simulink model "los_test_with_camsim_kalman2"  (Simulink 7.1)
settings: Solver=ode5  StartTime=0.0  StopTime=700  FixedStep=0.1  RelTol=1e-3
values from neighbouring files (symbols this model uses):
  bottom = u(7)    [camsim.m]    (also in camsim2.m = u(13); camsim3.m = u(13); ekf2.m = u(31); initauv.m = 4)
undefined symbols (not defined in the file or in its folder): ekf2
libraries: fordypningsprosjekt x3, simulink x1
settings Model: Creator=anderga  LastModifiedBy=anders

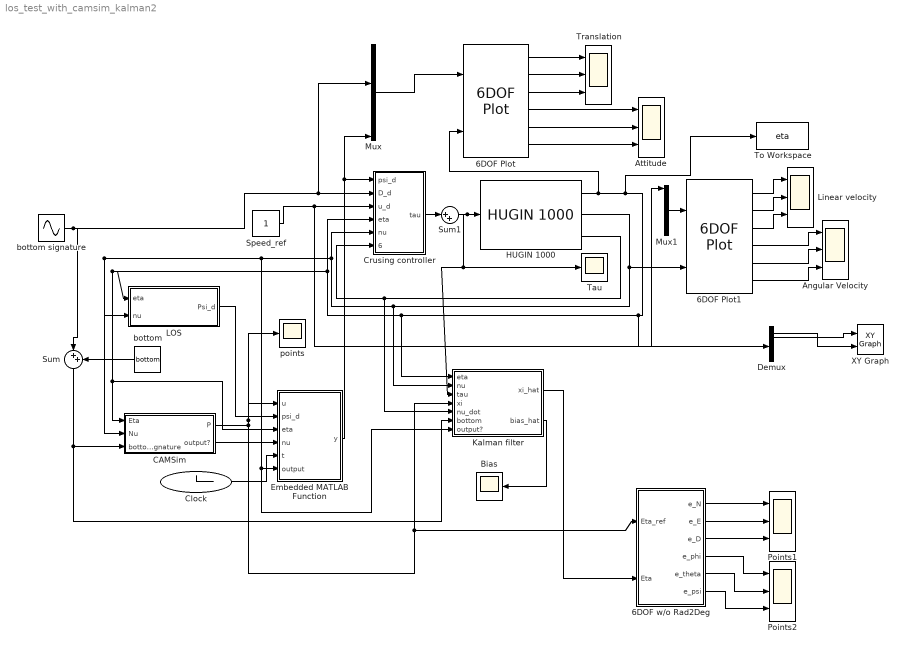
== system los_test_with_camsim_kalman2 ==
  6DOF Plot : fordypningsprosjekt/6DOF Plot  SystemSampleTime=-1
  6DOF Plot1 : fordypningsprosjekt/6DOF Plot  SystemSampleTime=-1
  6DOF w/o Rad2Deg : Subsystem  AncestorBlock=fordypningsprosjekt/6DOF Plot
      mask Type: 6 DOF plot reference versus eta
  Angular Velocity : Scope  NumInputPorts=3
      settings: YMin=-5~0~-40  YMax=5~0.3~40  SaveName=ScopeData3
  Attitude : Scope  NumInputPorts=3
      settings: YMin=-0.2~0~-200  YMax=0.25~0.5~200  SaveName=Attitude_ref
  Bias : Scope
      settings: YMin=-1  YMax=1  SaveName=Camsim_output1  DataFormat=Array
  CAMSim : Subsystem  AncestorBlock=fordypningsprosjekt/CAMSim
  Clock : Clock
  Crusing controller : Subsystem  AncestorBlock=fordypningsprosjekt/Crusing controller  mask{Kp_u=10, Ki_u=3, Kp_c=100, Kd_c=50, Kp_d=50, Kp2_d=20, Kd_d=20}
      mask prompts: Kp_u "Kp Speed controller"; Ki_u "Ki Speed Controller"; Kp_c "Kp Course Controller"; Kd_c "Kd Course Controller"; Kp_d "Kp1 Depth Controller"; Kp2_d "Kp2 Depth controller"; Kd_d "Kd Depth Controller"
  Demux : Demux  Outputs=6
  Embedded MATLAB Function : Stateflow chart
  HUGIN 1000 : fordypningsprosjekt/HUGIN 1000  SystemSampleTime=-1  eta_0=eta0  nu_0=[0 0 0 0 0 0]  c_on_off=off  beta_c=45  V_c=0.5
  Kalman filter : Subsystem  AncestorBlock=fordypningsprosjekt/Kalman filter
  LOS : Subsystem
  Linear velocity : Scope  NumInputPorts=3
      settings: YMin=0.5~-1.25~-0.125  YMax=1.9~0.75~0  SaveName=Lin_veloc
  Mux : Mux  Inputs=6
  Mux1 : Mux  Inputs=6
  Points1 : Scope  NumInputPorts=3
      settings: YMin=-1.75~-0.5~-1.75  YMax=0.5~0.5~0.5  SaveName=Translation_ref1
  Points2 : Scope  NumInputPorts=3
      settings: TimeRange=700  YMin=-0.4~-1.25~-0.5  YMax=0.5~0.5~0.5  SaveName=Attitude_ref1
  Speed_ref : Constant  OutDataType=sfix(16)  OutScaling=2^0
  Sum : Sum  Orientation=down  Inputs=|++  OutDataType=sfix(16)  OutScaling=2^0
  Sum1 : Sum  Inputs=|++  OutDataType=sfix(16)  OutScaling=2^0
  Tau : Scope
      settings: TimeRange=700  YMin=-5500  YMax=3000  SaveName=ScopeData4
  To Workspace : ToWorkspace  VariableName=eta  SampleTime=-1  SaveFormat=Structure With Time
  Translation : Scope  NumInputPorts=3
      settings: YMin=0~-125~0  YMax=125~0~60  SaveName=Translation_ref
  XY Graph : simulink/Sinks/XY Graph  SystemSampleTime=-1  xmin=-100  xmax=100  ymin=-100  ymax=500  st=-1
  bottom : Constant  Orientation=left  Value=bottom  OutDataType=sfix(16)  OutScaling=2^0
  bottom signature : Sin  Amplitude=6  Bias=50  Frequency=0.01  SampleTime=0
  points : Scope
      settings: TimeRange=500  YMin=-0.035  YMax=0.035  SaveName=Camsim_output  DataFormat=Array
  wires:
  HUGIN 1000/1 -> 6DOF Plot/2, Demux/1, Crusing controller/4(eta), LOS/1(eta), CAMSim/1(Eta), Embedded MATLAB Function/3(eta), Kalman filter/1(eta), To Workspace/1
  HUGIN 1000/2 -> 6DOF Plot1/2, Crusing controller/5(nu), LOS/2(nu), CAMSim/2(Nu), Embedded MATLAB Function/4(nu), Kalman filter/2(nu)
  HUGIN 1000/3 -> Crusing controller/6(nu_dot), Kalman filter/5(nu_dot)
  bottom signature/1 -> Crusing controller/2(D_d), Mux/3, Sum/1
  Speed_ref/1 -> Crusing controller/3(u_d), Mux1/1
  Mux/1 -> 6DOF Plot/1
  6DOF Plot/1 -> Translation/1
  6DOF Plot/2 -> Translation/2
  6DOF Plot/3 -> Translation/3
  6DOF Plot/4 -> Attitude/1
  6DOF Plot/5 -> Attitude/2
  6DOF Plot/6 -> Attitude/3
  Mux1/1 -> 6DOF Plot1/1
  6DOF Plot1/1 -> Linear velocity/1
  6DOF Plot1/2 -> Linear velocity/2
  6DOF Plot1/3 -> Linear velocity/3
  6DOF Plot1/4 -> Angular Velocity/1
  6DOF Plot1/5 -> Angular Velocity/2
  6DOF Plot1/6 -> Angular Velocity/3
  Demux/1 -> XY Graph/2
  Demux/2 -> XY Graph/1
  Sum/1 -> CAMSim/3(bottom_signature), Kalman filter/6(bottom)
  bottom/1 -> Sum/2
  Embedded MATLAB Function/1(y) -> Crusing controller/1(psi_d), Mux/6
  LOS/1(Psi_d) -> Embedded MATLAB Function/2(psi_d)
  CAMSim/1(P) -> Embedded MATLAB Function/1(u), points/1, 6DOF w/o Rad2Deg/1(Eta_ref), Kalman filter/4(xi)
  Clock/1 -> Embedded MATLAB Function/5(t)
  Kalman filter/1(xi_hat) -> 6DOF w/o Rad2Deg/2(Eta)
  6DOF w/o Rad2Deg/1(e_N) -> Points1/1
  6DOF w/o Rad2Deg/2(e_E) -> Points1/2
  6DOF w/o Rad2Deg/3(e_D) -> Points1/3
  6DOF w/o Rad2Deg/4(e_phi) -> Points2/1
  6DOF w/o Rad2Deg/5(e_theta) -> Points2/2
  6DOF w/o Rad2Deg/6(e_psi) -> Points2/3
  Kalman filter/2(bias_hat) -> Bias/1
  Crusing controller/1(tau) -> Sum1/1
  Sum1/1 -> HUGIN 1000/1, Tau/1, Kalman filter/3(tau)
  CAMSim/2(output?) -> Embedded MATLAB Function/6(output), Kalman filter/7(output?)

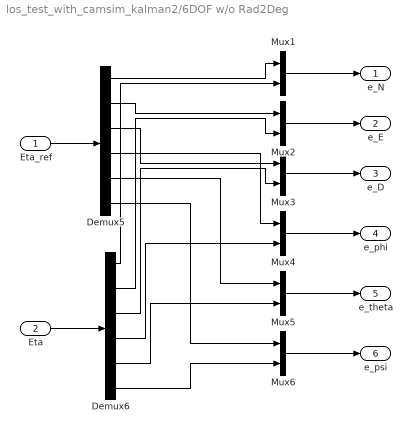
== system los_test_with_camsim_kalman2/6DOF w/o Rad2Deg ==
  Eta_ref : Inport  OutDataType=sfix(16)  OutScaling=2^0
  Eta : Inport  Port=2  OutDataType=sfix(16)  OutScaling=2^0
  Demux5 : Demux  Outputs=6
  Demux6 : Demux  Outputs=6
  Mux{1..6} (6 alike) : Mux  Inputs=2
  e_N : Outport  OutDataType=sfix(16)  OutScaling=2^0
  e_E : Outport  Port=2  OutDataType=sfix(16)  OutScaling=2^0
  e_D : Outport  Port=3  OutDataType=sfix(16)  OutScaling=2^0
  e_phi : Outport  Port=4  OutDataType=sfix(16)  OutScaling=2^0
  e_theta : Outport  Port=5  OutDataType=sfix(16)  OutScaling=2^0
  e_psi : Outport  Port=6  OutDataType=sfix(16)  OutScaling=2^0
  wires:
  Demux5/1 -> Mux1/1
  Demux6/1 -> Mux1/2
  Demux5/2 -> Mux2/1
  Demux5/3 -> Mux3/1
  Demux6/2 -> Mux2/2
  Demux6/3 -> Mux3/2
  Eta/1 -> Demux6/1
  Mux1/1 -> e_N/1
  Mux2/1 -> e_E/1
  Mux3/1 -> e_D/1
  Mux4/1 -> e_phi/1
  Mux5/1 -> e_theta/1
  Mux6/1 -> e_psi/1
  Demux5/4 -> Mux4/1
  Demux6/4 -> Mux4/2
  Demux5/5 -> Mux5/1
  Demux6/5 -> Mux5/2
  Demux6/6 -> Mux6/2
  Demux5/6 -> Mux6/1
  Eta_ref/1 -> Demux5/1

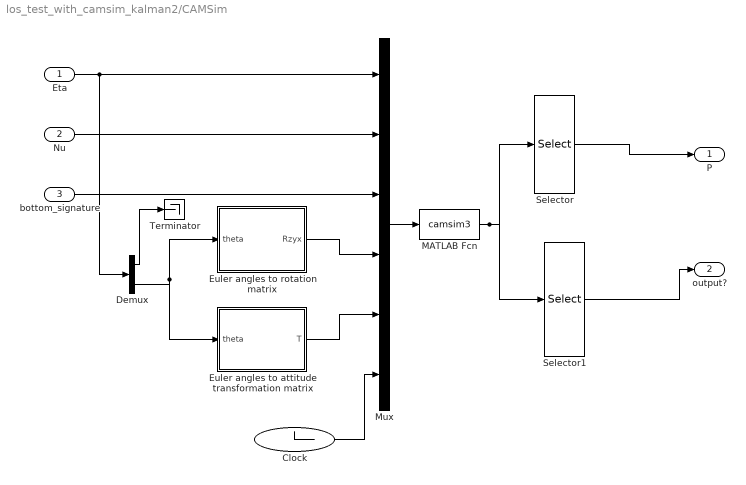
== system los_test_with_camsim_kalman2/CAMSim ==
  Eta : Inport  OutDataType=sfix(16)  OutScaling=2^0
  Nu : Inport  Port=2  OutDataType=sfix(16)  OutScaling=2^0
  bottom_signature : Inport  Port=3  OutDataType=sfix(16)  OutScaling=2^0
  Clock : Clock
  Demux : Demux  Outputs=2
  Euler angles to rotation matrix : Subsystem  AncestorBlock=marine_gnc/Models/ Kinematics/Euler angles to rotation matrix
      mask Type: Euler2R
      mask Description:
      | Determine the 3-by-3 rotation matrix from the Euler angles (roll, pitch, yaw) using the zyx convention.
      | 
      | Output is a 9x1 vector
      mask Display:
      | port_label('input',1,'theta')
      | port_label('output',1,'R')
  Euler angles to attitude transformation matrix : Subsystem  AncestorBlock=marine_gnc/Models/ Kinematics/Euler angles to attitude transformation matrix
      mask Type: Euler2T
      mask Description: Determine the 3-by-3 attitude transformation matrix  from the Euler angles (roll, pitch, yaw).
      mask Display:
      | port_label('input',1,'theta')
      | port_label('output',1,'T')
  MATLAB Fcn : MATLABFcn  MATLABFcn=camsim3  OutputDimensions=7
  Mux : Mux  Inputs=6
  Selector : Selector  InputPortWidth=7  IndexOptions=Index vector (dialog)  Indices=[1 2 3 4 5 6]  OutputSizes=1
  Selector1 : Selector  InputPortWidth=7  IndexOptions=Index vector (dialog)  Indices=[7]  OutputSizes=1
  Terminator : Terminator
  P : Outport  OutDataType=sfix(16)  OutScaling=2^0
  output? : Outport  Port=2  OutDataType=sfix(16)  OutScaling=2^0
  wires:
  Eta/1 -> Mux/1, Demux/1
  Nu/1 -> Mux/2
  bottom_signature/1 -> Mux/3
  Mux/1 -> MATLAB Fcn/1
  Demux/2 -> Euler angles to attitude transformation matrix/1(theta), Euler angles to rotation matrix/1(theta)
  Demux/1 -> Terminator/1
  Euler angles to rotation matrix/1(Rzyx) -> Mux/4
  Euler angles to attitude transformation matrix/1(T) -> Mux/5
  Clock/1 -> Mux/6
  MATLAB Fcn/1 -> Selector1/1, Selector/1
  Selector/1 -> P/1
  Selector1/1 -> output?/1

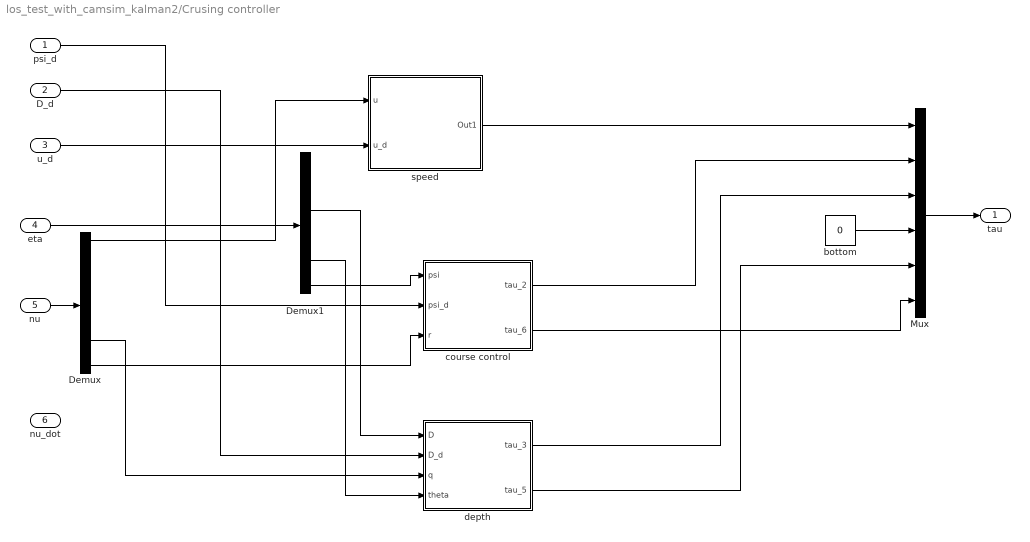
== system los_test_with_camsim_kalman2/Crusing controller ==
  psi_d : Inport  OutDataType=sfix(16)  OutScaling=2^0
  D_d : Inport  Port=2  OutDataType=sfix(16)  OutScaling=2^0
  u_d : Inport  Port=3  OutDataType=sfix(16)  OutScaling=2^0
  eta : Inport  Port=4  OutDataType=sfix(16)  OutScaling=2^0
  nu : Inport  Port=5  OutDataType=sfix(16)  OutScaling=2^0
  nu_dot : Inport  Port=6  OutDataType=sfix(16)  OutScaling=2^0
  Demux : Demux  Outputs=6
  Demux1 : Demux  Outputs=6
  Mux : Mux  Inputs=6
  bottom : Constant  Value=0  OutDataType=sfix(16)  OutScaling=2^0
  course control : Subsystem
  depth : Subsystem
  speed : Subsystem
  tau : Outport  OutDataType=sfix(16)  OutScaling=2^0
  wires:
  nu/1 -> Demux/1
  Demux/1 -> speed/1(u)
  u_d/1 -> speed/2(u_d)
  eta/1 -> Demux1/1
  Demux1/6 -> course control/1(psi)
  psi_d/1 -> course control/2(psi_d)
  Demux/6 -> course control/3(r)
  speed/1(Out1) -> Mux/1
  Mux/1 -> tau/1
  course control/1(tau_2) -> Mux/2
  course control/2(tau_6) -> Mux/6
  D_d/1 -> depth/2(D_d)
  Demux1/3 -> depth/1(D)
  Demux/5 -> depth/3(q)
  Demux1/5 -> depth/4(theta)
  depth/1(tau_3) -> Mux/3
  depth/2(tau_5) -> Mux/5
  bottom/1 -> Mux/4

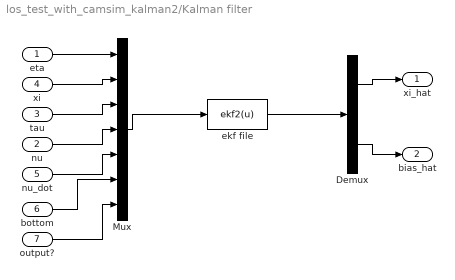
== system los_test_with_camsim_kalman2/Kalman filter ==
  eta : Inport  OutDataType=sfix(16)  OutScaling=2^0
  nu : Inport  Port=2  OutDataType=sfix(16)  OutScaling=2^0
  tau : Inport  Port=3  OutDataType=sfix(16)  OutScaling=2^0
  xi : Inport  Port=4  OutDataType=sfix(16)  OutScaling=2^0
  nu_dot : Inport  Port=5  OutDataType=sfix(16)  OutScaling=2^0
  bottom : Inport  Port=6  OutDataType=sfix(16)  OutScaling=2^0
  output? : Inport  Port=7  OutDataType=sfix(16)  OutScaling=2^0
  Demux : Demux  Outputs=2
  Mux : Mux  Inputs=7
  ekf file : MATLABFcn  MATLABFcn=ekf2(u)  OutputDimensions=12
  xi_hat : Outport  OutDataType=sfix(16)  OutScaling=2^0
  bias_hat : Outport  Port=2  OutDataType=sfix(16)  OutScaling=2^0
  wires:
  eta/1 -> Mux/1
  Mux/1 -> ekf file/1
  ekf file/1 -> Demux/1
  xi/1 -> Mux/2
  tau/1 -> Mux/3
  nu/1 -> Mux/4
  nu_dot/1 -> Mux/5
  bottom/1 -> Mux/6
  Demux/1 -> xi_hat/1
  Demux/2 -> bias_hat/1
  output?/1 -> Mux/7

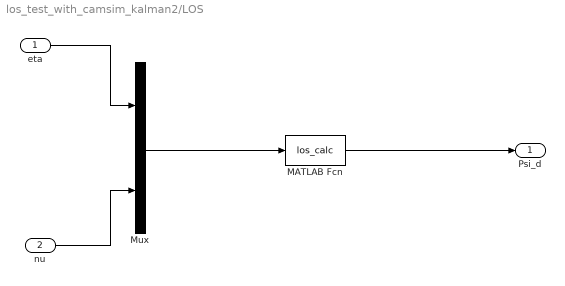
== system los_test_with_camsim_kalman2/LOS ==
  eta : Inport  OutDataType=sfix(16)  OutScaling=2^0
  nu : Inport  Port=2  OutDataType=sfix(16)  OutScaling=2^0
  MATLAB Fcn : MATLABFcn  MATLABFcn=los_calc  OutputDimensions=1
  Mux : Mux  Inputs=2
  Psi_d : Outport  OutDataType=sfix(16)  OutScaling=2^0
  wires:
  eta/1 -> Mux/1
  nu/1 -> Mux/2
  Mux/1 -> MATLAB Fcn/1
  MATLAB Fcn/1 -> Psi_d/1

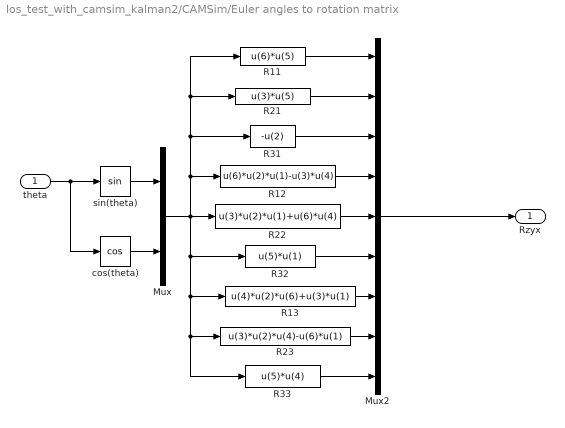
== system los_test_with_camsim_kalman2/CAMSim/Euler angles to rotation matrix ==
  theta : Inport  OutDataType=sfix(16)  OutScaling=2^0
  Mux : Mux  Inputs=2
  Mux2 : Mux  Inputs=9
  R11 : Fcn  Expr=u(6)*u(5)
  R12 : Fcn  Expr=u(6)*u(2)*u(1)-u(3)*u(4)
  R13 : Fcn  Expr=u(4)*u(2)*u(6)+u(3)*u(1)
  "R21 " : Fcn  Expr=u(3)*u(5)
  R22 : Fcn  Expr=u(3)*u(2)*u(1)+u(6)*u(4)
  R23 : Fcn  Expr=u(3)*u(2)*u(4)-u(6)*u(1)
  "R31 " : Fcn  Expr=-u(2)
  R32 : Fcn  Expr=u(5)*u(1)
  R33 : Fcn  Expr=u(5)*u(4)
  cos(theta) : Trigonometry  Operator=cos
  sin(theta) : Trigonometry
  Rzyx : Outport  OutDataType=sfix(16)  OutScaling=2^0  InitialOutput=0
  wires:
  R33/1 -> Mux2/9
  R32/1 -> Mux2/6
  "R21 "/1 -> Mux2/2
  "R31 "/1 -> Mux2/3
  R12/1 -> Mux2/4
  R22/1 -> Mux2/5
  R13/1 -> Mux2/7
  R23/1 -> Mux2/8
  Mux/1 -> R12/1, "R21 "/1, R11/1, "R31 "/1, R22/1, R23/1, R33/1, R13/1, R32/1
  theta/1 -> cos(theta)/1, sin(theta)/1
  cos(theta)/1 -> Mux/2
  sin(theta)/1 -> Mux/1
  Mux2/1 -> Rzyx/1
  R11/1 -> Mux2/1

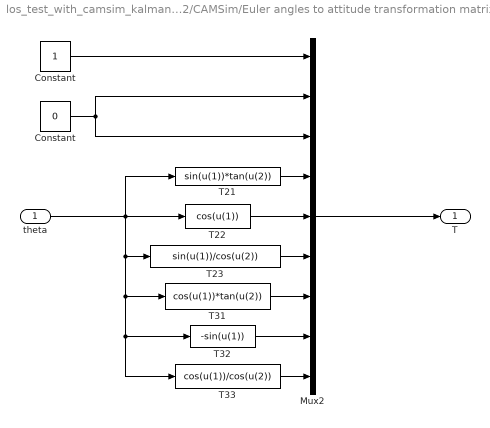
== system los_test_with_camsim_kalman2/CAMSim/Euler angles to attitude transformation matrix ==
  theta : Inport  OutDataType=sfix(16)  OutScaling=2^0
  Constant : Constant  OutDataType=sfix(16)  OutScaling=2^0
  "Constant " : Constant  Value=0  OutDataType=sfix(16)  OutScaling=2^0
  Mux2 : Mux  Inputs=9
  "T21 " : Fcn  Expr=sin(u(1))*tan(u(2))
  T22 : Fcn  Expr=cos(u(1))
  T23 : Fcn  Expr=sin(u(1))/cos(u(2))
  "T31 " : Fcn  Expr=cos(u(1))*tan(u(2))
  T32 : Fcn  Expr=-sin(u(1))
  T33 : Fcn  Expr=cos(u(1))/cos(u(2))
  T : Outport  OutDataType=sfix(16)  OutScaling=2^0  InitialOutput=0
  wires:
  T32/1 -> Mux2/8
  "T31 "/1 -> Mux2/7
  "T21 "/1 -> Mux2/4
  "Constant "/1 -> Mux2/3, Mux2/2
  T33/1 -> Mux2/9
  T22/1 -> Mux2/5
  T23/1 -> Mux2/6
  theta/1 -> "T21 "/1, T22/1, "T31 "/1, T32/1, T33/1, T23/1
  Mux2/1 -> T/1
  Constant/1 -> Mux2/1

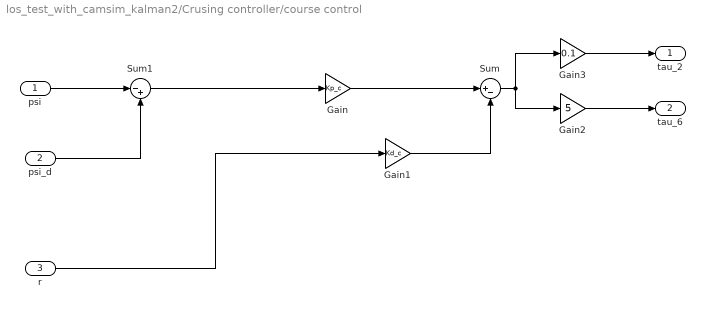
== system los_test_with_camsim_kalman2/Crusing controller/course control ==
  psi : Inport  OutDataType=sfix(16)  OutScaling=2^0
  psi_d : Inport  Port=2  OutDataType=sfix(16)  OutScaling=2^0
  r : Inport  Port=3  OutDataType=sfix(16)  OutScaling=2^0
  Gain : Gain  Gain=Kp_c  ParameterDataType=sfix(16)  ParameterScaling=2^0  OutDataType=sfix(16)  OutScaling=2^0
  Gain1 : Gain  Gain=Kd_c  ParameterDataType=sfix(16)  ParameterScaling=2^0  OutDataType=sfix(16)  OutScaling=2^0
  Gain2 : Gain  Gain=5  ParameterDataType=sfix(16)  ParameterScaling=2^0  OutDataType=sfix(16)  OutScaling=2^0
  Gain3 : Gain  Gain=0.1  ParameterDataType=sfix(16)  ParameterScaling=2^0  OutDataType=sfix(16)  OutScaling=2^0
  Sum : Sum  Inputs=|+-  OutDataType=sfix(16)  OutScaling=2^0
  Sum1 : Sum  Inputs=|-+  OutDataType=sfix(16)  OutScaling=2^0
  tau_2 : Outport  OutDataType=sfix(16)  OutScaling=2^0
  tau_6 : Outport  Port=2  OutDataType=sfix(16)  OutScaling=2^0
  wires:
  Sum1/1 -> Gain/1
  Gain1/1 -> Sum/2
  psi/1 -> Sum1/1
  psi_d/1 -> Sum1/2
  Gain/1 -> Sum/1
  r/1 -> Gain1/1
  Sum/1 -> Gain2/1, Gain3/1
  Gain2/1 -> tau_6/1
  Gain3/1 -> tau_2/1

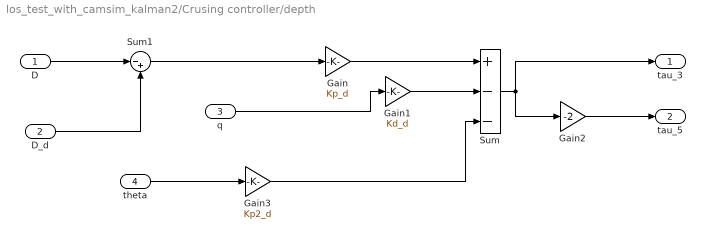
== system los_test_with_camsim_kalman2/Crusing controller/depth ==
  D : Inport  OutDataType=sfix(16)  OutScaling=2^0
  D_d : Inport  Port=2  OutDataType=sfix(16)  OutScaling=2^0
  q : Inport  Port=3  OutDataType=sfix(16)  OutScaling=2^0
  theta : Inport  Port=4  OutDataType=sfix(16)  OutScaling=2^0
  Gain : Gain  Gain=Kp_d  ParameterDataType=sfix(16)  ParameterScaling=2^0  OutDataType=sfix(16)  OutScaling=2^0
  Gain1 : Gain  Gain=Kd_d  ParameterDataType=sfix(16)  ParameterScaling=2^0  OutDataType=sfix(16)  OutScaling=2^0
  Gain2 : Gain  Gain=-2  ParameterDataType=sfix(16)  ParameterScaling=2^0  OutDataType=sfix(16)  OutScaling=2^0
  Gain3 : Gain  Gain=Kp2_d  ParameterDataType=sfix(16)  ParameterScaling=2^0  OutDataType=sfix(16)  OutScaling=2^0
  Sum : Sum  Inputs=+--  OutDataType=sfix(16)  OutScaling=2^0
  Sum1 : Sum  Inputs=|-+  OutDataType=sfix(16)  OutScaling=2^0
  tau_3 : Outport  OutDataType=sfix(16)  OutScaling=2^0
  tau_5 : Outport  Port=2  OutDataType=sfix(16)  OutScaling=2^0
  wires:
  Gain2/1 -> tau_5/1
  Sum/1 -> tau_3/1, Gain2/1
  q/1 -> Gain1/1
  Gain/1 -> Sum/1
  D_d/1 -> Sum1/2
  D/1 -> Sum1/1
  Gain1/1 -> Sum/2
  Sum1/1 -> Gain/1
  theta/1 -> Gain3/1
  Gain3/1 -> Sum/3

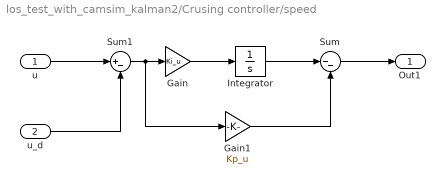
== system los_test_with_camsim_kalman2/Crusing controller/speed ==
  u : Inport  OutDataType=sfix(16)  OutScaling=2^0
  u_d : Inport  Port=2  OutDataType=sfix(16)  OutScaling=2^0
  Gain : Gain  Gain=Ki_u  ParameterDataType=sfix(16)  ParameterScaling=2^0  OutDataType=sfix(16)  OutScaling=2^0
  Gain1 : Gain  Gain=Kp_u  ParameterDataType=sfix(16)  ParameterScaling=2^0  OutDataType=sfix(16)  OutScaling=2^0
  Integrator : Integrator
  Sum : Sum  Inputs=|--  OutDataType=sfix(16)  OutScaling=2^0
  Sum1 : Sum  Inputs=|+-  OutDataType=sfix(16)  OutScaling=2^0
  Out1 : Outport  OutDataType=sfix(16)  OutScaling=2^0
  wires:
  Sum/1 -> Out1/1
  u/1 -> Sum1/1
  u_d/1 -> Sum1/2
  Sum1/1 -> Gain/1, Gain1/1
  Integrator/1 -> Sum/1
  Gain/1 -> Integrator/1
  Gain1/1 -> Sum/2

== matlab function Embedded MATLAB Function ==
  data: u input double; y output double; psi_d input double; eta input double; nu input double; t input double; output input double
function y = fcn(u, psi_d, eta , nu ,t, output)
% This block supports the Embedded MATLAB subset.
% See the help menu for details. 

persistent temp

if isempty(temp)
    temp = 0;
end

xi1 = u(1);
yi1 = u(2);
xi2 = u(3);
yi2 = u(4);
xi3 = u(5);
yi3 = u(6);

beta = atan2(nu(2), sqrt(nu(1)^2 + nu(2)^2));

    if output == 1    
        if xi1 >= eta(1)
            temp = atan2((yi1),(xi1)) + beta;
        else
            temp = atan2((yi3), (xi3)) + beta;
        end
     else
         temp = psi_d;  
    end   
    
y = temp;
